simulink model "Super9"  (Simulink 5.0)
settings: Solver=ode45  StartTime=0.0  StopTime=10.0  RelTol=1e-3
settings Model: Creator=scaife  LastModifiedBy=scaife  ExtModeAutoUpdateStatusClock=off

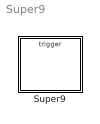
== system Super9 ==
  Super9 : Stateflow chart

== stateflow chart Super9 ==
  state A
  state B
    state B1
    state B2
    B1 -> B2 : E
  (default) -> A
  A -> B1 : E
  B2 -> A : E
  events: E input EITHER_EDGE_EVENT
